simulink model "sampleModel1918"  (R2023a)
settings: Solver=VariableStepAuto  StartTime=0.0  StopTime=10.0  RelTol=1e-3
libraries: hdlsllib x8, simulink x3
settings Model: Creator=user1  LastModifiedBy=user1

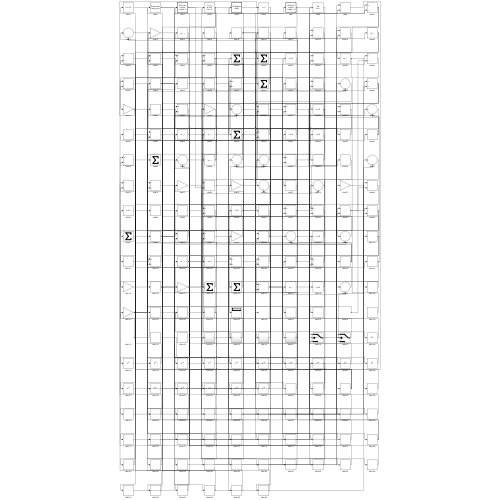
[thumbnail: Simulink's stored preview of the top-level diagram]
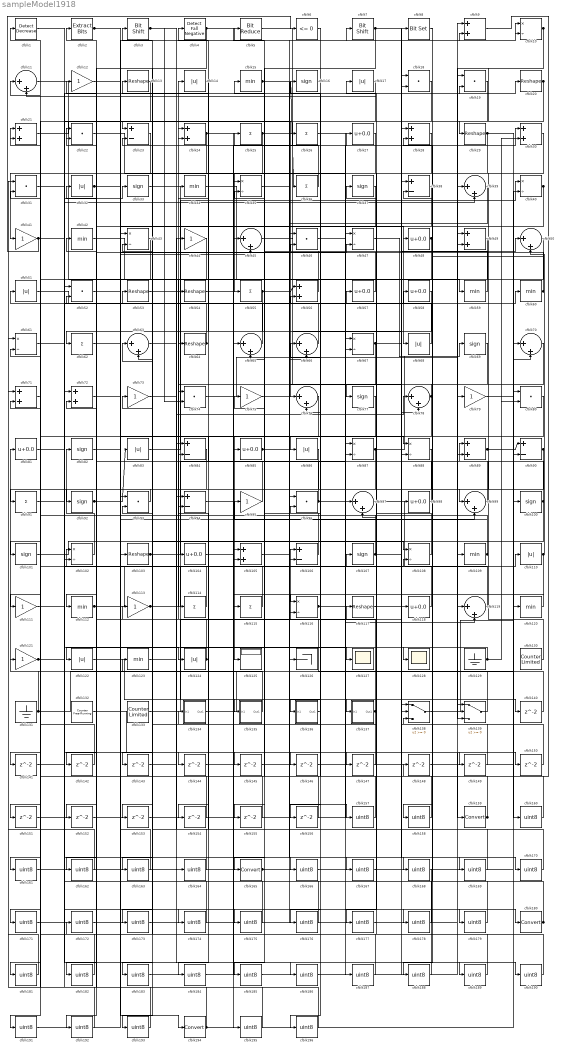
== system sampleModel1918 ==
  cfblk1 : simulink/Logic and Bit Operations/Detect Decrease  vinit=0.0  OutDataTypeStr=boolean
      settings: LibrarySourceBlock=|
      | hdlsllib/Logic and Bit
      | Operations/Detect
      | Decrease
  cfblk{10,35,40,43,47,61,67,87..88,102,108,116} (12 alike) : Product  Inputs=*/  RndMeth=Zero  SaturateOnIntegerOverflow=on
  cfblk{16,33,37,69,77,82,92,100..101,107} (10 alike) : Signum
  cfblk{13,20,29,53..54,64,103,117} (8 alike) : Reshape
  cfblk{27,48,57..58,81,85,98,104,118} (9 alike) : Bias  Bias=0.0  SaturateOnIntegerOverflow=off
  cfblk{9,21,24,28,30,49,56,71..72,89,105} (11 alike) : Sum
  cfblk{23,38,84,90,94,106} (6 alike) : Sum  Inputs=+-
  cfblk{15,34,42,59..60,109,112,120,123} (9 alike) : MinMax
  cfblk{11,39,45,50,63,65..66,70,76,78,97,99,119} (13 alike) : Sum  Inputs=|++
  cfblk{14,17,32,51,68,83,86,110,122,124} (10 alike) : Abs  SaturateOnIntegerOverflow=off
  cfblk{12,41,44,73,75,79,95,111,113,121} (10 alike) : Gain
  cfblk{25..26,36,55,62,91,114..115} (8 alike) : Sum  Inputs=+
  cfblk125 : Display
  cfblk126 : Terminator
  cfblk127 : Scope
  cfblk128 : Scope
  cfblk129 : Ground
  cfblk130 : hdlsllib/Sources/Counter Limited  uplimit=7  tsamp=-1
  cfblk131 : Ground
  cfblk132 : hdlsllib/Sources/Counter Free-Running  NumBits=16  tsamp=-1
  cfblk133 : hdlsllib/Sources/Counter Limited  uplimit=7  tsamp=-1
  cfblk134 : Subsystem
      settings: LibrarySourceBlock=|
      | hdlsllib/Ports &
      | Subsystems/Subsystem
  cfblk135 : Subsystem
      settings: LibrarySourceBlock=|
      | hdlsllib/Ports &
      | Subsystems/Subsystem
  cfblk136 : Subsystem
      settings: LibrarySourceBlock=|
      | hdlsllib/Ports &
      | Subsystems/Subsystem
  cfblk137 : Subsystem
      settings: LibrarySourceBlock=|
      | hdlsllib/Ports &
      | Subsystems/Subsystem
  cfblk138 : Switch  SaturateOnIntegerOverflow=off  InputSameDT=off
  cfblk139 : Switch  SaturateOnIntegerOverflow=off  InputSameDT=off
  cfblk{140..156} (17 alike) : Delay  SampleTime=1
  cfblk{157..158,160..164,166..179,181..193,195..196} (36 alike) : DataTypeConversion  OutDataTypeStr=uint8  SaturateOnIntegerOverflow=off  RndMeth=Floor
  cfblk{159,165,180,194} (4 alike) : DataTypeConversion  SaturateOnIntegerOverflow=off  RndMeth=Floor
  cfblk{18..19,22,31,46,52,74,80,93,96} (10 alike) : DotProduct  OutDataTypeStr=Inherit: Inherit via internal rule
  cfblk2 : simulink/Logic and Bit Operations/Extract Bits  bitsToExtract=Upper half  numBits=8  bitIdxRange=[0 7]  outScalingMode=Preserve fixed-point scaling
      settings: LibrarySourceBlock=|
      | hdlsllib/Logic and Bit
      | Operations/Extract Bits
  cfblk3 : hdlsllib/Logic and Bit Operations/Bit Shift  mode=Shift Left Logical  N=0
  cfblk4 : hdlsllib/Logic and Bit Operations/Detect Fall Negative  vinit=0  OutDataTypeStr=boolean
  cfblk5 : hdlsllib/Logic and Bit Operations/Bit Reduce  mode=AND
  cfblk6 : hdlsllib/Logic and Bit Operations/Compare To Zero  relop=<=  OutDataTypeStr=boolean
  cfblk7 : hdlsllib/Logic and Bit Operations/Bit Shift  mode=Shift Left Logical  N=0
  cfblk8 : simulink/Logic and Bit Operations/Bit Set  iBit=0
      settings: LibrarySourceBlock=|
      | hdlsllib/Logic and Bit
      | Operations/Bit Set
  wires:
  cfblk40/1 -> cfblk68/1, cfblk139/2, cfblk155/1
  cfblk39/1 -> cfblk76/1
  cfblk53/1 -> cfblk137/1(In1)
  cfblk77/1 -> cfblk125/1
  cfblk23/1 -> cfblk41/1
  cfblk64/1 -> cfblk13/1, cfblk54/1
  cfblk33/1 -> cfblk127/1
  cfblk102/1 -> cfblk82/1
  cfblk48/1 -> cfblk111/1, cfblk143/1
  cfblk25/1 -> cfblk55/1, cfblk88/2
  cfblk92/1 -> cfblk83/1, cfblk7/1, cfblk45/2
  cfblk113/1 -> cfblk107/1, cfblk78/1
  cfblk114/1 -> cfblk73/1
  cfblk47/1 -> cfblk69/1
  cfblk110/1 -> cfblk50/2, cfblk156/1
  cfblk90/1 -> cfblk161/1, cfblk185/1
  cfblk34/1 -> cfblk109/1
  cfblk124/1 -> cfblk14/1, cfblk184/1
  cfblk131/1 -> cfblk81/1, cfblk80/1
  cfblk83/1 -> cfblk40/1
  cfblk87/1 -> cfblk39/1, cfblk91/1
  cfblk42/1 -> cfblk114/1
  cfblk36/1 -> cfblk3/1
  cfblk45/1 -> cfblk77/1
  cfblk2/1 -> cfblk144/1, cfblk145/1
  cfblk3/1 -> cfblk84/1, cfblk74/2
  cfblk97/1 -> cfblk110/1
  cfblk30/1 -> cfblk99/1
  cfblk103/1 -> cfblk47/1, cfblk150/1
  cfblk136/1(Out1) -> cfblk66/1
  cfblk85/1 -> cfblk9/2, cfblk147/1
  cfblk11/1 -> cfblk119/1
  cfblk51/1 -> cfblk60/1
  cfblk74/1 -> cfblk9/1
  cfblk69/1 -> cfblk128/1
  cfblk106/1 -> cfblk15/1
  cfblk68/1 -> cfblk24/1
  cfblk133/1 -> cfblk8/1
  cfblk139/1 -> cfblk106/1
  cfblk5/1 -> cfblk138/1
  cfblk137/1(Out1) -> cfblk134/1(In1), cfblk102/1
  cfblk50/1 -> cfblk86/1
  cfblk41/1 -> cfblk6/1, cfblk170/1
  cfblk65/1 -> cfblk21/1
  cfblk14/1 -> cfblk64/1
  cfblk17/1 -> cfblk46/1
  cfblk119/1 -> cfblk51/1
  cfblk61/1 -> cfblk180/1
  cfblk37/1 -> cfblk116/1
  cfblk120/1 -> cfblk115/1
  cfblk138/1 -> cfblk100/1
  cfblk57/1 -> cfblk25/1
  cfblk93/1 -> cfblk92/1
  cfblk82/1 -> cfblk47/2
  cfblk91/1 -> cfblk124/1
  cfblk52/1 -> cfblk194/1
  cfblk7/1 -> cfblk45/1, cfblk169/1
  cfblk107/1 -> cfblk32/1, cfblk10/1
  cfblk20/1 -> cfblk76/2, cfblk102/2
  cfblk15/1 -> cfblk36/1, cfblk78/2
  cfblk4/1 -> cfblk10/2, cfblk173/1, cfblk192/1
  cfblk109/1 -> cfblk11/1, cfblk56/2, cfblk95/1
  cfblk19/1 -> cfblk65/2
  cfblk135/1(Out1) -> cfblk121/1
  cfblk59/1 -> cfblk37/1
  cfblk134/1(Out1) -> cfblk97/1
  cfblk60/1 -> cfblk12/1, cfblk38/2
  cfblk24/1 -> cfblk179/1, cfblk181/1
  cfblk1/1 -> cfblk26/1
  cfblk95/1 -> cfblk84/2
  cfblk105/1 -> cfblk19/2
  cfblk58/1 -> cfblk62/1
  cfblk100/1 -> cfblk4/1, cfblk193/1, cfblk196/1
  cfblk112/1 -> cfblk44/1, cfblk99/2, cfblk149/1
  cfblk132/1 -> cfblk159/1
  cfblk96/1 -> cfblk34/1, cfblk178/1
  cfblk70/1 -> cfblk165/1
  cfblk89/1 -> cfblk90/1, cfblk80/2
  cfblk46/1 -> cfblk67/1
  cfblk66/1 -> cfblk5/1
  cfblk122/1 -> cfblk135/1(In1)
  cfblk38/1 -> cfblk112/1
  cfblk78/1 -> cfblk74/1, cfblk153/1
  cfblk99/1 -> cfblk16/1
  cfblk129/1 -> cfblk122/1, cfblk30/2
  cfblk54/1 -> cfblk27/1
  cfblk101/1 -> cfblk104/1
  cfblk29/1 -> cfblk120/1, cfblk151/1
  cfblk81/1 -> cfblk33/1
  cfblk118/1 -> cfblk46/2
  cfblk111/1 -> cfblk39/2
  cfblk22/1 -> cfblk87/1
  cfblk32/1 -> cfblk108/1, cfblk88/1, cfblk59/1
  cfblk10/1 -> cfblk29/1, cfblk139/3
  cfblk62/1 -> cfblk57/1
  cfblk115/1 -> cfblk42/1
  cfblk121/1 -> cfblk20/1, cfblk58/1, cfblk108/2, cfblk190/1
  cfblk12/1 -> cfblk48/1
  cfblk21/1 -> cfblk23/1
  cfblk116/1 -> cfblk119/2, cfblk138/2, cfblk30/1
  cfblk16/1 -> cfblk136/1(In1)
  cfblk130/1 -> cfblk89/1
  cfblk27/1 -> cfblk116/2
  cfblk98/1 -> cfblk22/1
  cfblk108/1 -> cfblk11/2
  cfblk56/1 -> cfblk24/2
  cfblk67/1 -> cfblk105/1, cfblk50/1
  cfblk55/1 -> cfblk56/1, cfblk105/2, cfblk35/2
  cfblk44/1 -> cfblk101/1
  cfblk117/1 -> cfblk140/1
  cfblk140/1 -> cfblk19/1
  cfblk76/1 -> cfblk141/1
  cfblk13/1 -> cfblk142/1
  cfblk142/1 -> cfblk1/1
  cfblk144/1 -> cfblk65/1
  cfblk145/1 -> cfblk87/2
  cfblk31/1 -> cfblk146/1
  cfblk146/1 -> cfblk40/2
  cfblk147/1 -> cfblk93/2
  cfblk9/1 -> cfblk148/1
  cfblk149/1 -> cfblk38/1
  cfblk150/1 -> cfblk138/3
  cfblk151/1 -> cfblk67/2
  cfblk84/1 -> cfblk152/1
  cfblk152/1 -> cfblk106/2
  cfblk153/1 -> cfblk66/2
  cfblk80/1 -> cfblk154/1
  cfblk154/1 -> cfblk23/2
  cfblk155/1 -> cfblk21/2
  cfblk156/1 -> cfblk53/1
  cfblk75/1 -> cfblk157/1
  cfblk157/1 -> cfblk96/1
  cfblk8/1 -> cfblk158/1
  cfblk158/1 -> cfblk75/1
  cfblk159/1 -> cfblk96/2, cfblk22/2, cfblk113/1, cfblk97/2
  cfblk79/1 -> cfblk160/1
  cfblk160/1 -> cfblk31/2
  cfblk161/1 -> cfblk79/1
  cfblk43/1 -> cfblk162/1
  cfblk162/1 -> cfblk31/1
  cfblk88/1 -> cfblk163/1
  cfblk163/1 -> cfblk43/1
  cfblk73/1 -> cfblk164/1
  cfblk164/1 -> cfblk43/2
  cfblk165/1 -> cfblk89/2, cfblk98/1
  cfblk143/1 -> cfblk166/1
  cfblk166/1 -> cfblk70/1
  cfblk35/1 -> cfblk167/1
  cfblk167/1 -> cfblk70/2
  cfblk94/1 -> cfblk168/1
  cfblk169/1 -> cfblk94/1
  cfblk170/1 -> cfblk94/2
  cfblk18/1 -> cfblk171/1
  cfblk171/1 -> cfblk126/1
  cfblk168/1 -> cfblk172/1
  cfblk172/1 -> cfblk18/1
  cfblk173/1 -> cfblk18/2
  cfblk72/1 -> cfblk174/1
  cfblk174/1 -> cfblk93/1
  cfblk141/1 -> cfblk175/1
  cfblk175/1 -> cfblk72/1
  cfblk6/1 -> cfblk176/1
  cfblk176/1 -> cfblk72/2
  cfblk28/1 -> cfblk177/1
  cfblk177/1 -> cfblk139/1
  cfblk178/1 -> cfblk28/1
  cfblk179/1 -> cfblk28/2
  cfblk180/1 -> cfblk35/1, cfblk117/1
  cfblk181/1 -> cfblk61/1
  cfblk86/1 -> cfblk182/1
  cfblk182/1 -> cfblk61/2
  cfblk49/1 -> cfblk183/1
  cfblk183/1 -> cfblk85/1
  cfblk184/1 -> cfblk49/1
  cfblk185/1 -> cfblk49/2
  cfblk63/1 -> cfblk186/1
  cfblk186/1 -> cfblk118/1
  cfblk26/1 -> cfblk187/1
  cfblk187/1 -> cfblk63/1
  cfblk148/1 -> cfblk188/1
  cfblk188/1 -> cfblk63/2
  cfblk123/1 -> cfblk189/1
  cfblk189/1 -> cfblk17/1
  cfblk190/1 -> cfblk123/1
  cfblk71/1 -> cfblk191/1
  cfblk191/1 -> cfblk103/1
  cfblk192/1 -> cfblk71/1
  cfblk193/1 -> cfblk71/2
  cfblk194/1 -> cfblk90/2, cfblk2/1
  cfblk104/1 -> cfblk195/1
  cfblk195/1 -> cfblk52/1
  cfblk196/1 -> cfblk52/2

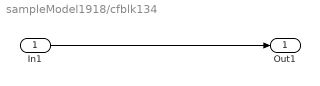
== system sampleModel1918/cfblk134 ==
  In1 : Inport
  Out1 : Outport
  wires:
  In1/1 -> Out1/1

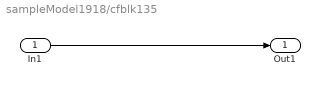
== system sampleModel1918/cfblk135 ==
  In1 : Inport
  Out1 : Outport
  wires:
  In1/1 -> Out1/1

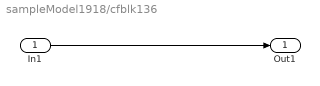
== system sampleModel1918/cfblk136 ==
  In1 : Inport
  Out1 : Outport
  wires:
  In1/1 -> Out1/1

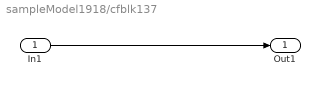
== system sampleModel1918/cfblk137 ==
  In1 : Inport
  Out1 : Outport
  wires:
  In1/1 -> Out1/1
